simulink model "UM7_SPI"  (R2018b)
settings: Solver=VariableStepAuto  StartTime=0.0  StopTime=10.0  RelTol=1e-3
values from neighbouring files (symbols this model uses):
  SPI_READ = [ ... (first row only)    [UM7.m]
libraries: c280xlib x2
settings Model: Creator=Syed Imtiaz Ali Shah  LastModifiedBy=Syed Imtiaz Ali Shah

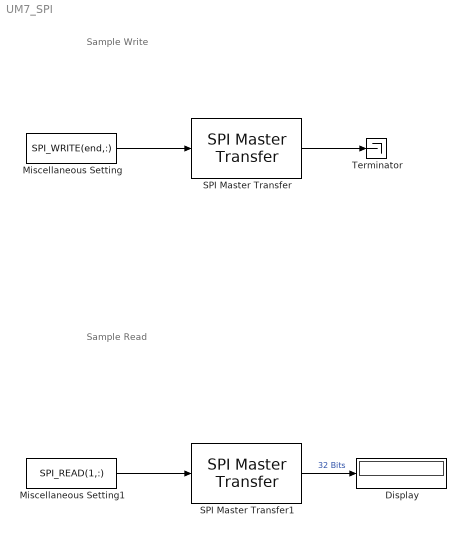
== system UM7_SPI ==
  note: Sample Write
  note: Sample Read
  Display : Display
  Miscellaneous Setting : Constant  Value=SPI_WRITE(end,:)  OutDataTypeStr=uint8
  Miscellaneous Setting1 : Constant  Value=SPI_READ(1,:)  OutDataTypeStr=uint8
  SPI Master Transfer : c280xlib/SPI Master Transfer  SPISelect=SPI_A  ClockPolarity=Rising_edge  ClockPhase=No_delay  SPIModule=uint32(0)  Mode=Master  BusSpeed=uint32(1000000)  FirstBitToTransfer=Most significant bit (MSB)  ClockMode=0  BlockFunction=Transfer  EnableRegisterAddress=on  RegisterAddress=0  OutputDataType=int8  OutputDataLength=1  DataBits=8  UseCustomSSPin=Provided by the SPI peripheral  ActiveLowSSPin=Active low  Pin=1
      settings: SourceProductName=Embedded Coder Support Package for Texas Instruments C2000 Processors  SourceProductBaseCode=TIC2000
  SPI Master Transfer1 : c280xlib/SPI Master Transfer  SPISelect=SPI_A  ClockPolarity=Rising_edge  ClockPhase=No_delay  SPIModule=uint32(0)  Mode=Master  BusSpeed=uint32(1000000)  FirstBitToTransfer=Most significant bit (MSB)  ClockMode=0  BlockFunction=Transfer  EnableRegisterAddress=on  RegisterAddress=0  OutputDataType=int8  OutputDataLength=1  DataBits=8  UseCustomSSPin=Provided by the SPI peripheral  ActiveLowSSPin=Active low  Pin=1
      settings: SourceProductName=Embedded Coder Support Package for Texas Instruments C2000 Processors  SourceProductBaseCode=TIC2000
  Terminator : Terminator
  wires:
  Miscellaneous Setting/1 -> SPI Master Transfer/1
  Miscellaneous Setting1/1 -> SPI Master Transfer1/1
  SPI Master Transfer/1 -> Terminator/1
  SPI Master Transfer1/1 -> Display/1  "32 Bits"
